simulink model "HemoDialysisMachine_Arch"  (R2023a)
settings: Solver=VariableStepAuto  StartTime=0.0  StopTime=3600*4  RelTol=1e-3
libraries: SignalEditorBlockLib x2
settings Model: Creator=ppatel  LastModifiedBy=ppatel
settings DebuggingCC: AlgebraicLoopMsg=none

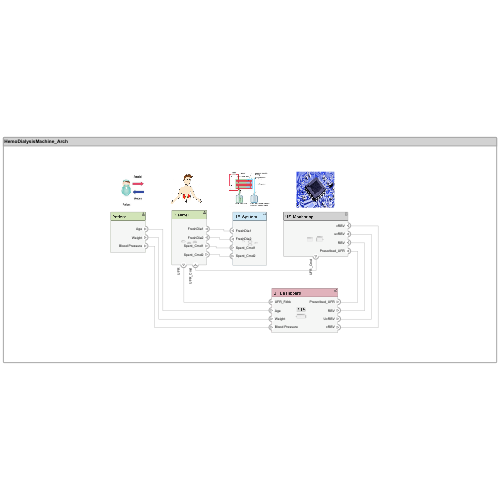
[thumbnail: Simulink's stored preview of the top-level diagram]
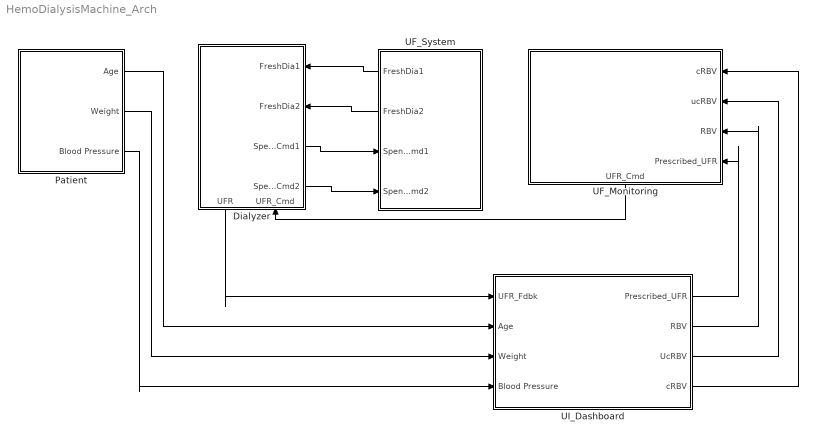
== system HemoDialysisMachine_Arch ==
  Dialyzer : Subsystem
      settings: PortSchema="{\"entries\":[{\"content\":{\"headerSize\":26,\"margin\":15,\"minimumSpacing\":25,\"sides\":[{\"content\":{},\"type\":\"ConnectorPlacement.EquallySpacedRectSide\",\"uuid\":\"646d2c69-fb26-4ce3-9a1c-87f27dc8a7c9\"},{\"content\":{\"connectorIds\":[\"In1\",\"In2\",\"Out1\",\"Out2\"],\"side\":\"RIGHT\"},\"type\":\"ConnectorPlacement.EquallySpacedRectSide\",\"uuid\":\"7346902f-f0ff-4e8d-8c8a-3cdeffc7661f\"},{\"content\":{\"side\":\"TOP\"},\"type\":\"ConnectorPlacement.EquallySpacedRectSide\",\"uuid\":\"ae1fdeb4-7a94-4e22-b0ba-9939a152f67f\"},{\"content\":{\"connectorIds\":[\"Out3\",\"In3\"],\"side\":\"BOTTOM\"},\"type\":\"ConnectorPlacement.EquallySpacedRectSide\",\"uuid\":\"fd631687-1978-4108-a79b-44a5b4b3e436\"}]},\"type\":\"ConnectorPlacement.EquallySpacedConnector\",\"uuid\":\"38b9a048-c643-4d7d-b16c-6a6e9025a495\"}],\"packageUris\":[\"http://schema.mathworks.com/mf0/Connector/R2020b\"],\"version\":\"1.0\"}"
  Patient : Subsystem
      settings: PortSchema="{\"entries\":[{\"content\":{\"headerSize\":26,\"margin\":15,\"minimumSpacing\":25,\"sides\":[{\"content\":{},\"type\":\"ConnectorPlacement.EquallySpacedRectSide\",\"uuid\":\"c448f8e9-f718-4d55-8ae9-400f94c3ed78\"},{\"content\":{\"connectorIds\":[\"Out2\",\"Out1\",\"Out3\"],\"side\":\"RIGHT\"},\"type\":\"ConnectorPlacement.EquallySpacedRectSide\",\"uuid\":\"ddea2424-6372-4e6c-88b3-edcc675d5c44\"},{\"content\":{\"side\":\"TOP\"},\"type\":\"ConnectorPlacement.EquallySpacedRectSide\",\"uuid\":\"5d354b5e-50bd-48d5-b50b-494e2a22bc78\"},{\"content\":{\"side\":\"BOTTOM\"},\"type\":\"ConnectorPlacement.EquallySpacedRectSide\",\"uuid\":\"88796682-fa10-4ce9-9062-498094082345\"}]},\"type\":\"ConnectorPlacement.EquallySpacedConnector\",\"uuid\":\"86ba679c-83d4-47d3-bf8e-52e917b1fb5f\"}],\"packageUris\":[\"http://schema.mathworks.com/mf0/Connector/R2020b\"],\"version\":\"1.0\"}"
  UF_Monitoring : Subsystem
      settings: PortSchema="{\"entries\":[{\"content\":{\"headerSize\":26,\"margin\":15,\"minimumSpacing\":25,\"sides\":[{\"content\":{},\"type\":\"ConnectorPlacement.EquallySpacedRectSide\",\"uuid\":\"c448f8e9-f718-4d55-8ae9-400f94c3ed78\"},{\"content\":{\"connectorIds\":[\"In2\",\"In3\",\"In1\",\"In4\"],\"side\":\"RIGHT\"},\"type\":\"ConnectorPlacement.EquallySpacedRectSide\",\"uuid\":\"ddea2424-6372-4e6c-88b3-edcc675d5c44\"},{\"content\":{\"side\":\"TOP\"},\"type\":\"ConnectorPlacement.EquallySpacedRectSide\",\"uuid\":\"5d354b5e-50bd-48d5-b50b-494e2a22bc78\"},{\"content\":{\"connectorIds\":[\"Out1\"],\"side\":\"BOTTOM\"},\"type\":\"ConnectorPlacement.EquallySpacedRectSide\",\"uuid\":\"50ece032-5537-489c-8a4a-ab4621a78d52\"}]},\"type\":\"ConnectorPlacement.EquallySpacedConnector\",\"uuid\":\"86ba679c-83d4-47d3-bf8e-52e917b1fb5f\"}],\"packageUris\":[\"http://schema.mathworks.com/mf0/Connector/R2020b\"],\"version\":\"1.0\"}"
  UF_System : Subsystem
      settings: PortSchema="{\"entries\":[{\"content\":{\"headerSize\":26,\"margin\":15,\"minimumSpacing\":25,\"sides\":[{\"content\":{\"connectorIds\":[\"Out1\",\"Out2\",\"In1\",\"In2\"]},\"type\":\"ConnectorPlacement.EquallySpacedRectSide\",\"uuid\":\"c448f8e9-f718-4d55-8ae9-400f94c3ed78\"},{\"content\":{\"side\":\"RIGHT\"},\"type\":\"ConnectorPlacement.EquallySpacedRectSide\",\"uuid\":\"ddea2424-6372-4e6c-88b3-edcc675d5c44\"},{\"content\":{\"side\":\"TOP\"},\"type\":\"ConnectorPlacement.EquallySpacedRectSide\",\"uuid\":\"5d354b5e-50bd-48d5-b50b-494e2a22bc78\"},{\"content\":{\"side\":\"BOTTOM\"},\"type\":\"ConnectorPlacement.EquallySpacedRectSide\",\"uuid\":\"db485aa5-56d5-4b4f-8c85-ef7ebb11d81c\"}]},\"type\":\"ConnectorPlacement.EquallySpacedConnector\",\"uuid\":\"86ba679c-83d4-47d3-bf8e-52e917b1fb5f\"}],\"packageUris\":[\"http://schema.mathworks.com/mf0/Connector/R2020b\"],\"version\":\"1.0\"}"
  UI_Dashboard : Subsystem
      settings: PortSchema="{\"entries\":[{\"content\":{\"headerSize\":26,\"margin\":15,\"minimumSpacing\":25,\"sides\":[{\"content\":{\"connectorIds\":[\"In1\",\"In2\",\"In3\",\"In4\"]},\"type\":\"ConnectorPlacement.EquallySpacedRectSide\",\"uuid\":\"c448f8e9-f718-4d55-8ae9-400f94c3ed78\"},{\"content\":{\"connectorIds\":[\"Out1\",\"Out2\",\"Out3\",\"Out4\"],\"side\":\"RIGHT\"},\"type\":\"ConnectorPlacement.EquallySpacedRectSide\",\"uuid\":\"ddea2424-6372-4e6c-88b3-edcc675d5c44\"},{\"content\":{\"side\":\"TOP\"},\"type\":\"ConnectorPlacement.EquallySpacedRectSide\",\"uuid\":\"5d354b5e-50bd-48d5-b50b-494e2a22bc78\"}]},\"type\":\"ConnectorPlacement.EquallySpacedConnector\",\"uuid\":\"86ba679c-83d4-47d3-bf8e-52e917b1fb5f\"}],\"packageUris\":[\"http://schema.mathworks.com/mf0/Connector/R2020b\"],\"version\":\"1.0\"}"
  wires:
  Patient/1(Weight) -> UI_Dashboard/3(Weight)
  Patient/2(Age) -> UI_Dashboard/2(Age)
  Patient/3(Blood Pressure) -> UI_Dashboard/4(Blood Pressure)
  UI_Dashboard/1(Prescribed_UFR) -> UF_Monitoring/4(Prescribed_UFR)
  UI_Dashboard/2(RBV) -> UF_Monitoring/1(RBV)
  UI_Dashboard/3(UcRBV) -> UF_Monitoring/3(ucRBV)
  UI_Dashboard/4(cRBV) -> UF_Monitoring/2(cRBV)
  UF_Monitoring/1(UFR_Cmd) -> Dialyzer/3(UFR_Cmd)
  Dialyzer/3(UFR) -> UI_Dashboard/1(UFR_Fdbk)
  UF_System/1(FreshDia1) -> Dialyzer/1(FreshDia1)
  UF_System/2(FreshDia2) -> Dialyzer/2(FreshDia2)
  Dialyzer/1(Spent_Cmd1) -> UF_System/1(Spent_Cmd1)
  Dialyzer/2(Spent_Cmd2) -> UF_System/2(Spent_Cmd2)

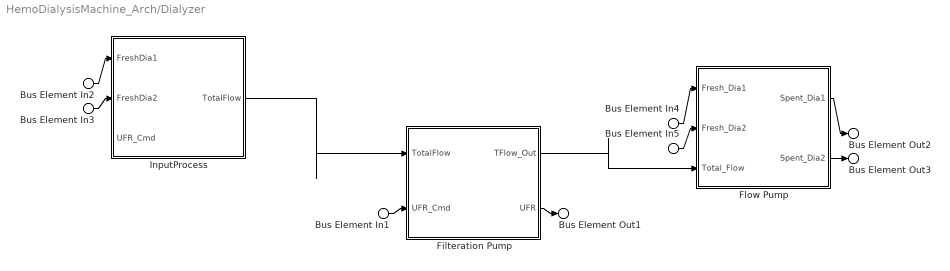
== system HemoDialysisMachine_Arch/Dialyzer ==
  Bus Element In2 : Inport  PortName=FreshDia1
  Bus Element In4 : Inport  PortName=FreshDia1
  Bus Element In3 : Inport  Port=2  PortName=FreshDia2
  Bus Element In5 : Inport  Port=2  PortName=FreshDia2
  Bus Element In1 : Inport  Port=3  PortName=UFR_Cmd
  Filteration Pump : Subsystem  Variant=on  VariantControlMode=label  LabelModeActiveChoice=false
      settings: PortSchema="{\"entries\":[{\"content\":{\"headerSize\":38,\"margin\":15,\"minimumSpacing\":25,\"sides\":[{\"content\":{\"connectorIds\":[\"In1\",\"In2\"]},\"type\":\"ConnectorPlacement.EquallySpacedRectSide\",\"uuid\":\"9dabf490-3af2-45d6-8c60-cb1a1321c83a\"},{\"content\":{\"connectorIds\":[\"Out1\",\"Out2\"],\"side\":\"RIGHT\"},\"type\":\"ConnectorPlacement.EquallySpacedRectSide\",\"uuid\":\"a9747e4f-9c1f-4b08-97d0-3540262e7855\"},{\"content\":{\"side\":\"TOP\"},\"type\":\"ConnectorPlacement.EquallySpacedRectSide\",\"uuid\":\"69b7741e-5af4-4aec-bdfa-c21327b02f85\"}]},\"type\":\"ConnectorPlacement.EquallySpacedConnector\",\"uuid\":\"ef3de475-85da-4577-91ef-81f0604493ee\"}],\"packageUris\":[\"http://schema.mathworks.com/mf0/Connector/R2020b\"],\"version\":\"1.0\"}"
  Flow Pump : Subsystem  Variant=on  VariantControlMode=label  LabelModeActiveChoice=true
      settings: PortSchema="{\"entries\":[{\"content\":{\"headerSize\":38,\"margin\":15,\"minimumSpacing\":25,\"sides\":[{\"content\":{\"connectorIds\":[\"In1\",\"In2\",\"In3\"]},\"type\":\"ConnectorPlacement.EquallySpacedRectSide\",\"uuid\":\"9dabf490-3af2-45d6-8c60-cb1a1321c83a\"},{\"content\":{\"connectorIds\":[\"Out1\",\"Out2\"],\"side\":\"RIGHT\"},\"type\":\"ConnectorPlacement.EquallySpacedRectSide\",\"uuid\":\"a9747e4f-9c1f-4b08-97d0-3540262e7855\"},{\"content\":{\"side\":\"TOP\"},\"type\":\"ConnectorPlacement.EquallySpacedRectSide\",\"uuid\":\"69b7741e-5af4-4aec-bdfa-c21327b02f85\"}]},\"type\":\"ConnectorPlacement.EquallySpacedConnector\",\"uuid\":\"ef3de475-85da-4577-91ef-81f0604493ee\"}],\"packageUris\":[\"http://schema.mathworks.com/mf0/Connector/R2020b\"],\"version\":\"1.0\"}"
  InputProcess : Subsystem
      settings: PortSchema="{\"entries\":[{\"content\":{\"headerSize\":26,\"margin\":15,\"minimumSpacing\":25,\"sides\":[{\"content\":{\"connectorIds\":[\"In1\",\"In2\",\"In3\"]},\"type\":\"ConnectorPlacement.EquallySpacedRectSide\",\"uuid\":\"646d2c69-fb26-4ce3-9a1c-87f27dc8a7c9\"},{\"content\":{\"connectorIds\":[\"Out1\"],\"side\":\"RIGHT\"},\"type\":\"ConnectorPlacement.EquallySpacedRectSide\",\"uuid\":\"7346902f-f0ff-4e8d-8c8a-3cdeffc7661f\"},{\"content\":{\"side\":\"TOP\"},\"type\":\"ConnectorPlacement.EquallySpacedRectSide\",\"uuid\":\"ae1fdeb4-7a94-4e22-b0ba-9939a152f67f\"}]},\"type\":\"ConnectorPlacement.EquallySpacedConnector\",\"uuid\":\"38b9a048-c643-4d7d-b16c-6a6e9025a495\"}],\"packageUris\":[\"http://schema.mathworks.com/mf0/Connector/R2020b\"],\"version\":\"1.0\"}"
  Bus Element Out2 : Outport  PortName=Spent_Cmd1
  Bus Element Out3 : Outport  Port=2  PortName=Spent_Cmd2
  Bus Element Out1 : Outport  Port=3  PortName=UFR
  wires:
  InputProcess/1(TotalFlow) -> Filteration Pump/1(TotalFlow)
  Bus Element In1/1 -> Filteration Pump/2(UFR_Cmd)
  Filteration Pump/2(UFR) -> Bus Element Out1/1
  Filteration Pump/1(TFlow_Out) -> Flow Pump/3(Total_Flow)
  Bus Element In2/1 -> InputProcess/1(FreshDia1)
  Bus Element In3/1 -> InputProcess/2(FreshDia2)
  Bus Element In4/1 -> Flow Pump/1(Fresh_Dia1)
  Bus Element In5/1 -> Flow Pump/2(Fresh_Dia2)
  Flow Pump/1(Spent_Dia1) -> Bus Element Out2/1
  Flow Pump/2(Spent_Dia2) -> Bus Element Out3/1

== system HemoDialysisMachine_Arch/Patient ==
  Bus Element Out1 : Outport  PortName=Weight
  Bus Element Out2 : Outport  Port=2  PortName=Age
  Bus Element Out3 : Outport  Port=3  PortName=Blood Pressure

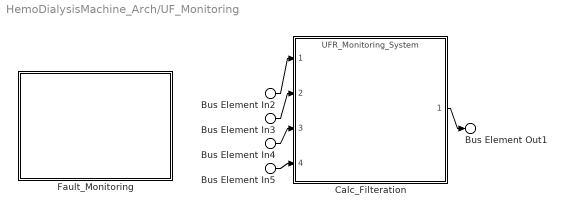
== system HemoDialysisMachine_Arch/UF_Monitoring ==
  Bus Element In3 : Inport  PortName=RBV
  Bus Element In4 : Inport  Port=2  PortName=cRBV
  Bus Element In5 : Inport  Port=3  PortName=ucRBV
  Bus Element In2 : Inport  Port=4  PortName=Prescribed_UFR
  Calc_Filteration : ModelReference  ModelNameDialog=UFR_Monitoring_System  SimulationMode=Normal  ModelReferenceVersion=3.74
      settings: PortSchema="{\"entries\":[{\"content\":{\"headerSize\":38,\"margin\":15,\"minimumSpacing\":25,\"sides\":[{\"content\":{\"connectorIds\":[\"In1\",\"In2\",\"In3\",\"In4\"]},\"type\":\"ConnectorPlacement.EquallySpacedRectSide\",\"uuid\":\"c448f8e9-f718-4d55-8ae9-400f94c3ed78\"},{\"content\":{\"connectorIds\":[\"Out1\"],\"side\":\"RIGHT\"},\"type\":\"ConnectorPlacement.EquallySpacedRectSide\",\"uuid\":\"ddea2424-6372-4e6c-88b3-edcc675d5c44\"},{\"content\":{\"side\":\"TOP\"},\"type\":\"ConnectorPlacement.EquallySpacedRectSide\",\"uuid\":\"5d354b5e-50bd-48d5-b50b-494e2a22bc78\"}]},\"type\":\"ConnectorPlacement.EquallySpacedConnector\",\"uuid\":\"86ba679c-83d4-47d3-bf8e-52e917b1fb5f\"}],\"packageUris\":[\"http://schema.mathworks.com/mf0/Connector/R2020b\"],\"version\":\"1.0\"}"
  Fault_Monitoring : Subsystem
      settings: PortSchema="{\"entries\":[{\"content\":{\"headerSize\":26,\"margin\":15,\"minimumSpacing\":25,\"sides\":[{\"content\":{},\"type\":\"ConnectorPlacement.EquallySpacedRectSide\",\"uuid\":\"a687e012-4840-413d-ae7b-c05f2b55ca05\"},{\"content\":{\"side\":\"RIGHT\"},\"type\":\"ConnectorPlacement.EquallySpacedRectSide\",\"uuid\":\"6a695777-1bf4-4cf6-ae1b-4fd6cbf201ea\"},{\"content\":{\"side\":\"TOP\"},\"type\":\"ConnectorPlacement.EquallySpacedRectSide\",\"uuid\":\"4e0efd68-4a3d-4565-a916-e6cda3743f29\"}]},\"type\":\"ConnectorPlacement.EquallySpacedConnector\",\"uuid\":\"de7bea47-d1da-4071-a467-1cf916758324\"}],\"packageUris\":[\"http://schema.mathworks.com/mf0/Connector/R2020b\"],\"version\":\"1.0\"}"
  Bus Element Out1 : Outport  PortName=UFR_Cmd
  wires:
  Bus Element In3/1 -> Calc_Filteration/2
  Bus Element In4/1 -> Calc_Filteration/3
  Bus Element In5/1 -> Calc_Filteration/4
  Bus Element In2/1 -> Calc_Filteration/1
  Calc_Filteration/1 -> Bus Element Out1/1

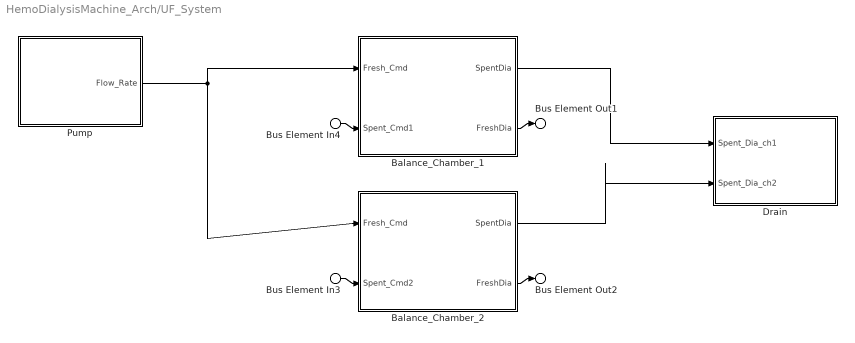
== system HemoDialysisMachine_Arch/UF_System ==
  Bus Element In4 : Inport  PortName=Spent_Cmd1
  Bus Element In3 : Inport  Port=2  PortName=Spent_Cmd2
  Balance_Chamber_1 : Subsystem
      settings: PortSchema="{\"entries\":[{\"content\":{\"headerSize\":26,\"margin\":15,\"minimumSpacing\":25,\"sides\":[{\"content\":{\"connectorIds\":[\"In1\",\"In2\"]},\"type\":\"ConnectorPlacement.EquallySpacedRectSide\",\"uuid\":\"c448f8e9-f718-4d55-8ae9-400f94c3ed78\"},{\"content\":{\"connectorIds\":[\"Out1\",\"Out2\"],\"side\":\"RIGHT\"},\"type\":\"ConnectorPlacement.EquallySpacedRectSide\",\"uuid\":\"ddea2424-6372-4e6c-88b3-edcc675d5c44\"},{\"content\":{\"side\":\"TOP\"},\"type\":\"ConnectorPlacement.EquallySpacedRectSide\",\"uuid\":\"5d354b5e-50bd-48d5-b50b-494e2a22bc78\"}]},\"type\":\"ConnectorPlacement.EquallySpacedConnector\",\"uuid\":\"86ba679c-83d4-47d3-bf8e-52e917b1fb5f\"}],\"packageUris\":[\"http://schema.mathworks.com/mf0/Connector/R2020b\"],\"version\":\"1.0\"}"
  Balance_Chamber_2 : Subsystem
      settings: PortSchema="{\"entries\":[{\"content\":{\"headerSize\":26,\"margin\":15,\"minimumSpacing\":25,\"sides\":[{\"content\":{\"connectorIds\":[\"In1\",\"In2\"]},\"type\":\"ConnectorPlacement.EquallySpacedRectSide\",\"uuid\":\"c448f8e9-f718-4d55-8ae9-400f94c3ed78\"},{\"content\":{\"connectorIds\":[\"Out1\",\"Out2\"],\"side\":\"RIGHT\"},\"type\":\"ConnectorPlacement.EquallySpacedRectSide\",\"uuid\":\"ddea2424-6372-4e6c-88b3-edcc675d5c44\"},{\"content\":{\"side\":\"TOP\"},\"type\":\"ConnectorPlacement.EquallySpacedRectSide\",\"uuid\":\"5d354b5e-50bd-48d5-b50b-494e2a22bc78\"}]},\"type\":\"ConnectorPlacement.EquallySpacedConnector\",\"uuid\":\"86ba679c-83d4-47d3-bf8e-52e917b1fb5f\"}],\"packageUris\":[\"http://schema.mathworks.com/mf0/Connector/R2020b\"],\"version\":\"1.0\"}"
  Drain : Subsystem
      settings: PortSchema="{\"entries\":[{\"content\":{\"headerSize\":26,\"margin\":15,\"minimumSpacing\":25,\"sides\":[{\"content\":{\"connectorIds\":[\"In1\",\"In2\"]},\"type\":\"ConnectorPlacement.EquallySpacedRectSide\",\"uuid\":\"c448f8e9-f718-4d55-8ae9-400f94c3ed78\"},{\"content\":{\"side\":\"RIGHT\"},\"type\":\"ConnectorPlacement.EquallySpacedRectSide\",\"uuid\":\"ddea2424-6372-4e6c-88b3-edcc675d5c44\"},{\"content\":{\"side\":\"TOP\"},\"type\":\"ConnectorPlacement.EquallySpacedRectSide\",\"uuid\":\"5d354b5e-50bd-48d5-b50b-494e2a22bc78\"}]},\"type\":\"ConnectorPlacement.EquallySpacedConnector\",\"uuid\":\"86ba679c-83d4-47d3-bf8e-52e917b1fb5f\"}],\"packageUris\":[\"http://schema.mathworks.com/mf0/Connector/R2020b\"],\"version\":\"1.0\"}"
  Pump : Subsystem
      settings: PortSchema="{\"entries\":[{\"content\":{\"headerSize\":26,\"margin\":15,\"minimumSpacing\":25,\"sides\":[{\"content\":{},\"type\":\"ConnectorPlacement.EquallySpacedRectSide\",\"uuid\":\"c448f8e9-f718-4d55-8ae9-400f94c3ed78\"},{\"content\":{\"connectorIds\":[\"Out1\"],\"side\":\"RIGHT\"},\"type\":\"ConnectorPlacement.EquallySpacedRectSide\",\"uuid\":\"ddea2424-6372-4e6c-88b3-edcc675d5c44\"},{\"content\":{\"side\":\"TOP\"},\"type\":\"ConnectorPlacement.EquallySpacedRectSide\",\"uuid\":\"5d354b5e-50bd-48d5-b50b-494e2a22bc78\"}]},\"type\":\"ConnectorPlacement.EquallySpacedConnector\",\"uuid\":\"86ba679c-83d4-47d3-bf8e-52e917b1fb5f\"}],\"packageUris\":[\"http://schema.mathworks.com/mf0/Connector/R2020b\"],\"version\":\"1.0\"}"
  Bus Element Out1 : Outport  PortName=FreshDia1
  Bus Element Out2 : Outport  Port=2  PortName=FreshDia2
  wires:
  Balance_Chamber_1/1(SpentDia) -> Drain/1(Spent_Dia_ch1)
  Balance_Chamber_2/1(SpentDia) -> Drain/2(Spent_Dia_ch2)
  Balance_Chamber_1/2(FreshDia) -> Bus Element Out1/1
  Balance_Chamber_2/2(FreshDia) -> Bus Element Out2/1
  Pump/1(Flow_Rate) -> Balance_Chamber_1/1(Fresh_Cmd), Balance_Chamber_2/1(Fresh_Cmd)
  Bus Element In3/1 -> Balance_Chamber_2/2(Spent_Cmd2)
  Bus Element In4/1 -> Balance_Chamber_1/2(Spent_Cmd1)

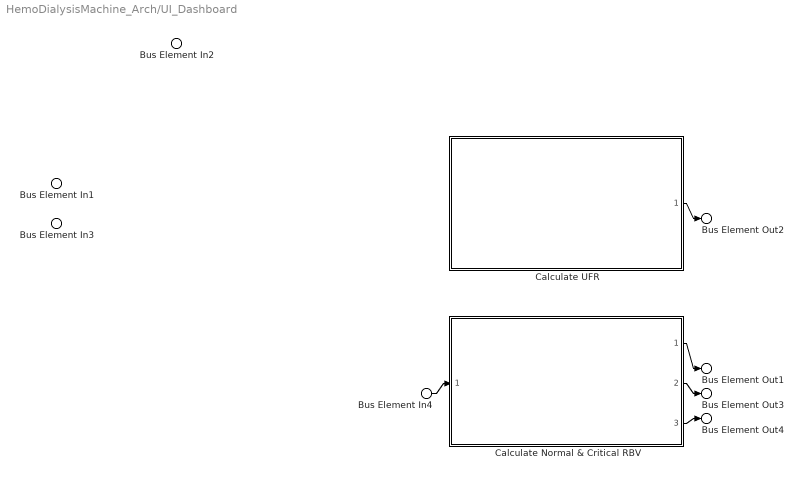
== system HemoDialysisMachine_Arch/UI_Dashboard ==
  Bus Element In4 : Inport  PortName=UFR_Fdbk
  Bus Element In2 : Inport  Port=2  PortName=Age
  Bus Element In1 : Inport  Port=3  PortName=Weight
  Bus Element In3 : Inport  Port=4  PortName=Blood Pressure
  Calculate Normal & Critical RBV : Subsystem  ReferencedSubsystem=CalculateNormalCriticalRBV
      settings: PortSchema="{\"entries\":[{\"content\":{\"headerSize\":26,\"margin\":15,\"minimumSpacing\":25,\"sides\":[{\"content\":{\"connectorIds\":[\"In1\"]},\"type\":\"ConnectorPlacement.EquallySpacedRectSide\",\"uuid\":\"646d2c69-fb26-4ce3-9a1c-87f27dc8a7c9\"},{\"content\":{\"connectorIds\":[\"Out1\",\"Out2\",\"Out3\"],\"side\":\"RIGHT\"},\"type\":\"ConnectorPlacement.EquallySpacedRectSide\",\"uuid\":\"7346902f-f0ff-4e8d-8c8a-3cdeffc7661f\"},{\"content\":{\"side\":\"TOP\"},\"type\":\"ConnectorPlacement.EquallySpacedRectSide\",\"uuid\":\"ae1fdeb4-7a94-4e22-b0ba-9939a152f67f\"}]},\"type\":\"ConnectorPlacement.EquallySpacedConnector\",\"uuid\":\"38b9a048-c643-4d7d-b16c-6a6e9025a495\"}],\"packageUris\":[\"http://schema.mathworks.com/mf0/Connector/R2020b\"],\"version\":\"1.0\"}"
  Calculate UFR : Subsystem  ReferencedSubsystem=Calculate_Prescribed_UFR  predw=73.2  postdw=70.6  dtime=4
      settings: PortSchema="{\"entries\":[{\"content\":{\"headerSize\":26,\"margin\":15,\"minimumSpacing\":25,\"sides\":[{\"content\":{},\"type\":\"ConnectorPlacement.EquallySpacedRectSide\",\"uuid\":\"646d2c69-fb26-4ce3-9a1c-87f27dc8a7c9\"},{\"content\":{\"connectorIds\":[\"Out1\"],\"side\":\"RIGHT\"},\"type\":\"ConnectorPlacement.EquallySpacedRectSide\",\"uuid\":\"7346902f-f0ff-4e8d-8c8a-3cdeffc7661f\"},{\"content\":{\"side\":\"TOP\"},\"type\":\"ConnectorPlacement.EquallySpacedRectSide\",\"uuid\":\"ae1fdeb4-7a94-4e22-b0ba-9939a152f67f\"}]},\"type\":\"ConnectorPlacement.EquallySpacedConnector\",\"uuid\":\"38b9a048-c643-4d7d-b16c-6a6e9025a495\"}],\"packageUris\":[\"http://schema.mathworks.com/mf0/Connector/R2020b\"],\"version\":\"1.0\"}"
  Bus Element Out2 : Outport  PortName=Prescribed_UFR
  Bus Element Out1 : Outport  Port=2  PortName=RBV
  Bus Element Out3 : Outport  Port=3  PortName=UcRBV
  Bus Element Out4 : Outport  Port=4  PortName=cRBV
  wires:
  Calculate UFR/1 -> Bus Element Out2/1
  Calculate Normal & Critical RBV/1 -> Bus Element Out1/1
  Calculate Normal & Critical RBV/2 -> Bus Element Out3/1
  Calculate Normal & Critical RBV/3 -> Bus Element Out4/1
  Bus Element In4/1 -> Calculate Normal & Critical RBV/1

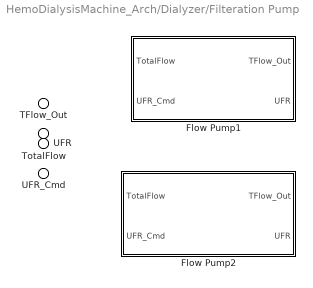
== system HemoDialysisMachine_Arch/Dialyzer/Filteration Pump ==
  TotalFlow : Inport
  UFR_Cmd : Inport  Port=2
  Flow Pump1 : Subsystem  VariantControl=true
      settings: PortSchema="{\"entries\":[{\"content\":{\"headerSize\":26,\"margin\":15,\"minimumSpacing\":25,\"sides\":[{\"content\":{\"connectorIds\":[\"In1\",\"In2\"]},\"type\":\"ConnectorPlacement.EquallySpacedRectSide\",\"uuid\":\"d349afe6-09cd-4458-bff5-c9b0512ae125\"},{\"content\":{\"connectorIds\":[\"Out1\",\"Out2\"],\"side\":\"RIGHT\"},\"type\":\"ConnectorPlacement.EquallySpacedRectSide\",\"uuid\":\"419f3d35-5a25-43f9-91a3-664932055dc6\"},{\"content\":{\"side\":\"TOP\"},\"type\":\"ConnectorPlacement.EquallySpacedRectSide\",\"uuid\":\"50db7389-90d3-44ed-82ed-d4679f63d180\"}]},\"type\":\"ConnectorPlacement.EquallySpacedConnector\",\"uuid\":\"cbfe1293-9b0f-4693-a82b-97c78c5df62e\"}],\"packageUris\":[\"http://schema.mathworks.com/mf0/Connector/R2020b\"],\"version\":\"1.0\"}"
  Flow Pump2 : Subsystem  VariantControl=false
      settings: PortSchema="{\"entries\":[{\"content\":{\"headerSize\":26,\"margin\":15,\"minimumSpacing\":25,\"sides\":[{\"content\":{\"connectorIds\":[\"In1\",\"In2\"]},\"type\":\"ConnectorPlacement.EquallySpacedRectSide\",\"uuid\":\"d349afe6-09cd-4458-bff5-c9b0512ae125\"},{\"content\":{\"connectorIds\":[\"Out1\",\"Out2\"],\"side\":\"RIGHT\"},\"type\":\"ConnectorPlacement.EquallySpacedRectSide\",\"uuid\":\"419f3d35-5a25-43f9-91a3-664932055dc6\"},{\"content\":{\"side\":\"TOP\"},\"type\":\"ConnectorPlacement.EquallySpacedRectSide\",\"uuid\":\"50db7389-90d3-44ed-82ed-d4679f63d180\"}]},\"type\":\"ConnectorPlacement.EquallySpacedConnector\",\"uuid\":\"cbfe1293-9b0f-4693-a82b-97c78c5df62e\"}],\"packageUris\":[\"http://schema.mathworks.com/mf0/Connector/R2020b\"],\"version\":\"1.0\"}"
  TFlow_Out : Outport
  UFR : Outport  Port=2

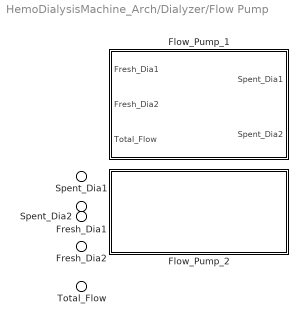
== system HemoDialysisMachine_Arch/Dialyzer/Flow Pump ==
  Fresh_Dia1 : Inport
  Fresh_Dia2 : Inport  Port=2
  Total_Flow : Inport  Port=3
  Flow_Pump_1 : Subsystem  VariantControl=true
      settings: PortSchema="{\"entries\":[{\"content\":{\"headerSize\":26,\"margin\":15,\"minimumSpacing\":25,\"sides\":[{\"content\":{\"connectorIds\":[\"In1\",\"In2\",\"In3\"]},\"type\":\"ConnectorPlacement.EquallySpacedRectSide\",\"uuid\":\"d349afe6-09cd-4458-bff5-c9b0512ae125\"},{\"content\":{\"connectorIds\":[\"Out1\",\"Out2\"],\"side\":\"RIGHT\"},\"type\":\"ConnectorPlacement.EquallySpacedRectSide\",\"uuid\":\"419f3d35-5a25-43f9-91a3-664932055dc6\"},{\"content\":{\"side\":\"TOP\"},\"type\":\"ConnectorPlacement.EquallySpacedRectSide\",\"uuid\":\"50db7389-90d3-44ed-82ed-d4679f63d180\"}]},\"type\":\"ConnectorPlacement.EquallySpacedConnector\",\"uuid\":\"cbfe1293-9b0f-4693-a82b-97c78c5df62e\"}],\"packageUris\":[\"http://schema.mathworks.com/mf0/Connector/R2020b\"],\"version\":\"1.0\"}"
  Flow_Pump_2 : Subsystem  VariantControl=false
      settings: PortSchema="{\"entries\":[{\"content\":{\"headerSize\":26,\"margin\":15,\"minimumSpacing\":25,\"sides\":[{\"content\":{},\"type\":\"ConnectorPlacement.EquallySpacedRectSide\",\"uuid\":\"d349afe6-09cd-4458-bff5-c9b0512ae125\"},{\"content\":{\"side\":\"RIGHT\"},\"type\":\"ConnectorPlacement.EquallySpacedRectSide\",\"uuid\":\"419f3d35-5a25-43f9-91a3-664932055dc6\"},{\"content\":{\"side\":\"TOP\"},\"type\":\"ConnectorPlacement.EquallySpacedRectSide\",\"uuid\":\"50db7389-90d3-44ed-82ed-d4679f63d180\"}]},\"type\":\"ConnectorPlacement.EquallySpacedConnector\",\"uuid\":\"cbfe1293-9b0f-4693-a82b-97c78c5df62e\"}],\"packageUris\":[\"http://schema.mathworks.com/mf0/Connector/R2020b\"],\"version\":\"1.0\"}"
  Spent_Dia1 : Outport
  Spent_Dia2 : Outport  Port=2

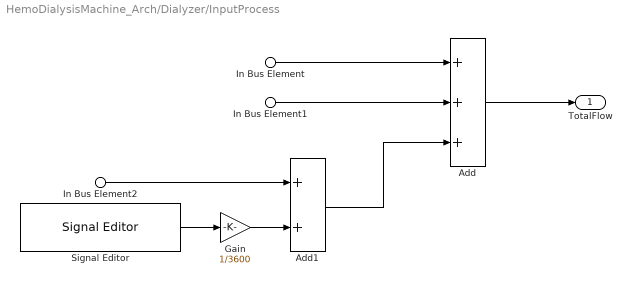
== system HemoDialysisMachine_Arch/Dialyzer/InputProcess ==
  In Bus Element : Inport  PortName=FreshDia1
  In Bus Element1 : Inport  Port=2  PortName=FreshDia2
  In Bus Element2 : Inport  Port=3  PortName=UFR_Cmd
  Add : Sum  Inputs=+++
  Add1 : Sum
  Gain : Gain  Gain=1/3600
  Signal Editor : SignalEditorBlockLib/Signal Editor  FileName=dialysisDemo_noise.mat  ActiveScenario=UltrafiltrationRate  ActiveSignal=UFR Noise (ml/hr)  IsBus=off  OutputBusObjectStr=Bus: BusObject  SampleTime=0  Interpolate=off  ZeroCross=off  OutputAfterFinalValue=Setting to zero  Unit=inherit  PreserveSignalName=on  ApplySigPropsToAllScenarios=on
  TotalFlow : Outport
  wires:
  In Bus Element/1 -> Add/1
  In Bus Element1/1 -> Add/2
  Signal Editor/1 -> Gain/1
  Gain/1 -> Add1/2
  In Bus Element2/1 -> Add1/1
  Add1/1 -> Add/3
  Add/1 -> TotalFlow/1

== system HemoDialysisMachine_Arch/UF_Monitoring/Fault_Monitoring ==

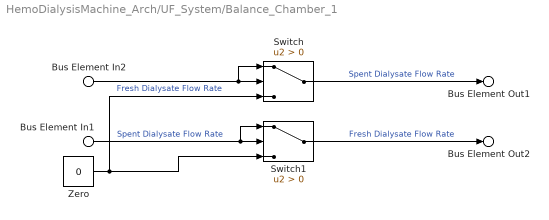
== system HemoDialysisMachine_Arch/UF_System/Balance_Chamber_1 ==
  Bus Element In2 : Inport  PortName=Fresh_Cmd
  Bus Element In1 : Inport  Port=2  PortName=Spent_Cmd1
  Switch : Switch  Criteria=u2 > Threshold  SaturateOnIntegerOverflow=off  InputSameDT=off
  Switch1 : Switch  Criteria=u2 > Threshold  SaturateOnIntegerOverflow=off  InputSameDT=off
  Zero : Constant  Value=0  OutDataTypeStr=Inherit: Inherit via back propagation
  Bus Element Out1 : Outport  PortName=SpentDia
  Bus Element Out2 : Outport  Port=2  PortName=FreshDia
  wires:
  Bus Element In1/1 -> Switch1/2, Switch1/1  "Spent Dialysate Flow Rate"
  Bus Element In2/1 -> Switch/2, Switch/1  "Fresh Dialysate Flow Rate"
  Switch1/1 -> Bus Element Out2/1  "Fresh Dialysate Flow Rate"
  Switch/1 -> Bus Element Out1/1  "Spent Dialysate Flow Rate"
  Zero/1 -> Switch/3, Switch1/3

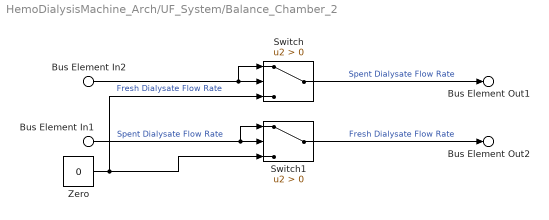
== system HemoDialysisMachine_Arch/UF_System/Balance_Chamber_2 ==
  Bus Element In2 : Inport  PortName=Fresh_Cmd
  Bus Element In1 : Inport  Port=2  PortName=Spent_Cmd2
  Switch : Switch  Criteria=u2 > Threshold  SaturateOnIntegerOverflow=off  InputSameDT=off
  Switch1 : Switch  Criteria=u2 > Threshold  SaturateOnIntegerOverflow=off  InputSameDT=off
  Zero : Constant  Value=0  OutDataTypeStr=Inherit: Inherit via back propagation
  Bus Element Out1 : Outport  PortName=SpentDia
  Bus Element Out2 : Outport  Port=2  PortName=FreshDia
  wires:
  Bus Element In1/1 -> Switch1/2, Switch1/1  "Spent Dialysate Flow Rate"
  Zero/1 -> Switch/3, Switch1/3
  Switch1/1 -> Bus Element Out2/1  "Fresh Dialysate Flow Rate"
  Bus Element In2/1 -> Switch/2, Switch/1  "Fresh Dialysate Flow Rate"
  Switch/1 -> Bus Element Out1/1  "Spent Dialysate Flow Rate"

== system HemoDialysisMachine_Arch/UF_System/Drain ==
  Bus Element In1 : Inport  PortName=Spent_Dia_ch1
  Bus Element In2 : Inport  Port=2  PortName=Spent_Dia_ch2

== system HemoDialysisMachine_Arch/UF_System/Pump ==
  Chart : Stateflow chart  TreatAsAtomicUnit=on
  Constant : Constant  Value=30000
  Display : Display
  Scope : Scope
  Bus Element Out1 : Outport  PortName=Flow_Rate
  wires:
  Constant/1 -> Chart/1(UFR), Display/1  "Ultrafiltration Rate"
  Chart/1(DFR_fresh) -> Bus Element Out1/1, Scope/1  "Fresh Dialysate Flow Rate"

== system HemoDialysisMachine_Arch/Dialyzer/Filteration Pump/Flow Pump1 ==
  Bus Element In1 : Inport  PortName=TotalFlow
  Bus Element In2 : Inport  Port=2  PortName=UFR_Cmd
  Bus Element Out1 : Outport  PortName=TFlow_Out
  Bus Element Out2 : Outport  Port=2  PortName=UFR

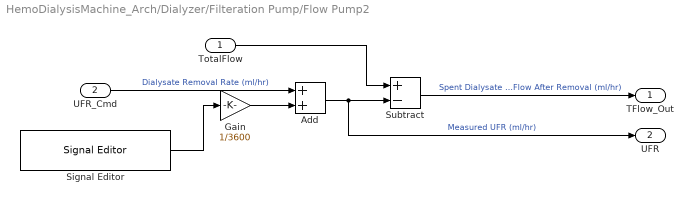
== system HemoDialysisMachine_Arch/Dialyzer/Filteration Pump/Flow Pump2 ==
  TotalFlow : Inport
  UFR_Cmd : Inport  Port=2
  Add : Sum
  Gain : Gain  Gain=1/3600
  Signal Editor : SignalEditorBlockLib/Signal Editor  FileName=dialysisDemo_noise.mat  ActiveScenario=UltrafiltratePump  ActiveSignal=UF Pump Noise (ml/hr)  IsBus=off  OutputBusObjectStr=Bus: BusObject  SampleTime=0  Interpolate=off  ZeroCross=off  OutputAfterFinalValue=Setting to zero  Unit=inherit  PreserveSignalName=on  ApplySigPropsToAllScenarios=on
  Subtract : Sum  Inputs=+-
  TFlow_Out : Outport
  UFR : Outport  Port=2
  wires:
  Subtract/1 -> TFlow_Out/1  "Spent Dialysate Flow After Removal (ml/hr)"
  UFR_Cmd/1 -> Add/1  "Dialysate Removal Rate (ml/hr)"
  Signal Editor/1 -> Gain/1
  TotalFlow/1 -> Subtract/1
  Add/1 -> Subtract/2, UFR/1  "Measured UFR (ml/hr)"
  Gain/1 -> Add/2

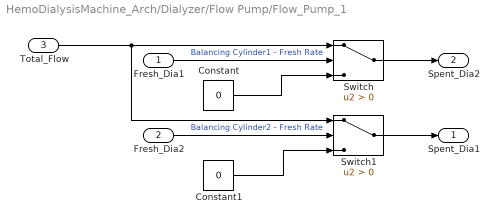
== system HemoDialysisMachine_Arch/Dialyzer/Flow Pump/Flow_Pump_1 ==
  Fresh_Dia1 : Inport
  Fresh_Dia2 : Inport  Port=2
  Total_Flow : Inport  Port=3
  Constant : Constant  Value=0  SampleTime=-1
  Constant1 : Constant  Value=0  SampleTime=-1
  Switch : Switch  Criteria=u2 > Threshold  SaturateOnIntegerOverflow=off  InputSameDT=off
  Switch1 : Switch  Criteria=u2 > Threshold  SaturateOnIntegerOverflow=off  InputSameDT=off
  Spent_Dia1 : Outport
  Spent_Dia2 : Outport  Port=2
  wires:
  Total_Flow/1 -> Switch1/1, Switch/1
  Constant/1 -> Switch/3
  Constant1/1 -> Switch1/3
  Switch/1 -> Spent_Dia2/1
  Fresh_Dia2/1 -> Switch1/2  "Balancing Cylinder2 - Fresh Rate"
  Switch1/1 -> Spent_Dia1/1
  Fresh_Dia1/1 -> Switch/2  "Balancing Cylinder1 - Fresh Rate"

== system HemoDialysisMachine_Arch/Dialyzer/Flow Pump/Flow_Pump_2 ==

== stateflow chart HemoDialysisMachine_Arch/UF_System/Pump/Chart ==
  state FillCylinder2
    entry: DFR_fresh = [UFR, 0];
    during: DFR_fresh = [UFR, 0];
  state FillCylinder1
    entry: DFR_fresh = [0, UFR];
    during: DFR_fresh = [0, UFR];
  (default) -> FillCylinder1
  FillCylinder2 -> FillCylinder1 : after(30*3600/UFR, sec)
  FillCylinder1 -> FillCylinder2 : after(30*3600/UFR, sec)
  data: UFR input; DFR_fresh output
